simulink model "Tema7_Slink"  (R2014a)
settings: Solver=ode45  StartTime=0.0  StopTime=10.0  RelTol=1e-3
libraries: cstblocks x3, simulink x1
settings Model: Creator=giova  LastModifiedBy=giova

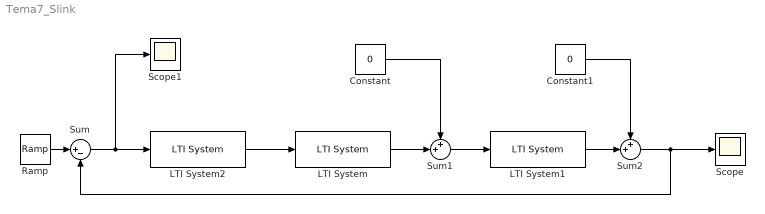
== system Tema7_Slink ==
  Constant : Constant  Value=0
  Constant1 : Constant  Value=0
  LTI System : cstblocks/LTI System  sys=F1  IC=[]
  LTI System1 : cstblocks/LTI System  sys=F2  IC=[]
  LTI System2 : cstblocks/LTI System  sys=C  IC=[]
  Ramp : simulink/Sources/Ramp  slope=1  start=0  X0=0
  Scope : Scope
  Scope1 : Scope
      settings: TimeRange=10  YMin=0  YMax=0.14
  Sum : Sum  Inputs=|+-
  Sum1 : Sum  Inputs=++|
  Sum2 : Sum  Inputs=++|
  wires:
  LTI System2/1 -> LTI System/1
  Sum/1 -> Scope1/1, LTI System2/1
  LTI System/1 -> Sum1/2
  Sum1/1 -> LTI System1/1
  LTI System1/1 -> Sum2/2
  Sum2/1 -> Scope/1, Sum/2
  Ramp/1 -> Sum/1
  Constant1/1 -> Sum2/1
  Constant/1 -> Sum1/1
